simulink subsystem "rss_MotoStallDiaHybr"  (R2023a)
settings: Solver=VariableStepAuto  StartTime=0.0  StopTime=10.0  RelTol=1e-3
undefined symbols (not defined in the file): Cdbl_nElecAgSpdMaxVal, Cdbl_psiPermMagFlxMaxVal, Cdbl_psiPermMagFlxMinVal, ENM_AG_POS_EVAL_MODE, ENM_TYPE_FALT, Gs16_nMotoStallMinRefElecSpd_C, Gu16_ctMotoStallConfCnt_C, Gu16_ctMotoStallRcvyCnt_C, Gu16_psiEstMinPermMagFlx_C
libraries: lib_debounce x1, simulink x1, lib_fault_definiteness x1
settings Model: Creator=xiaoqiang.yuan  LastModifiedBy=xiaoqiang.yuan

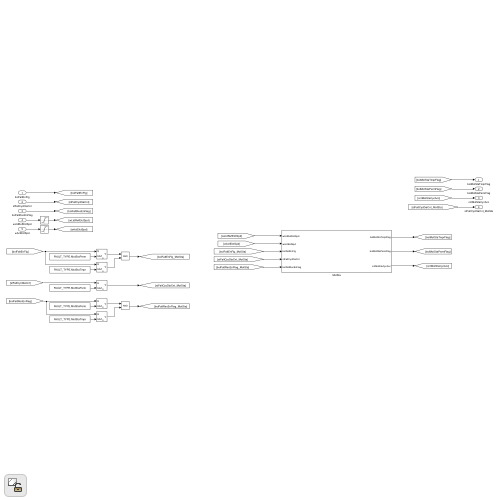
[thumbnail: Simulink's stored preview of the top-level diagram]
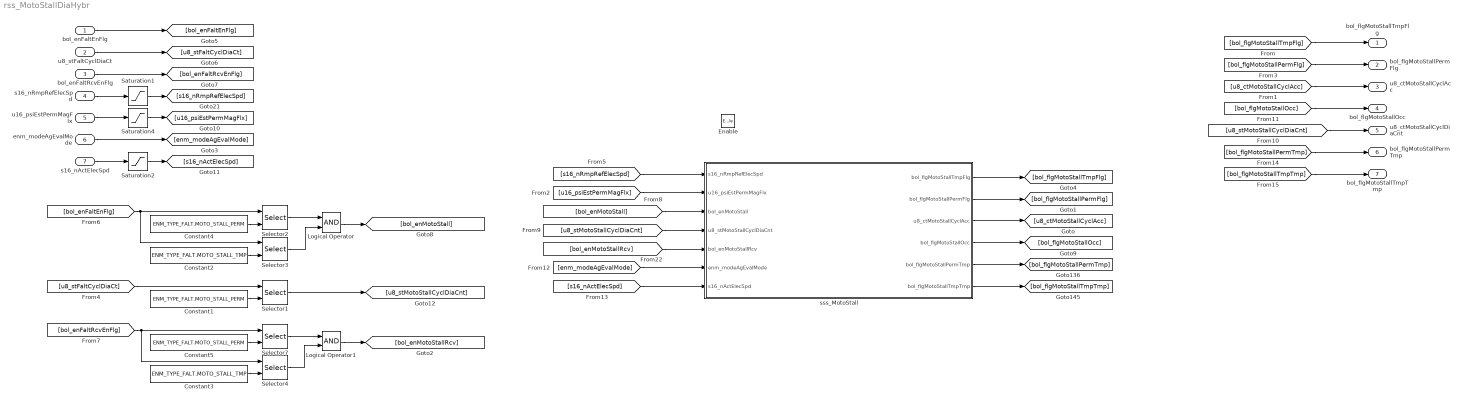
== system rss_MotoStallDiaHybr ==
  bol_enFaltEnFlg : Inport  OutDataTypeStr=boolean
  u8_stFaltCyclDiaCt : Inport  Port=2  OutDataTypeStr=uint8
  bol_enFaltRcvEnFlg : Inport  Port=3  OutDataTypeStr=boolean
  s16_nRmpRefElecSpd : Inport  Port=4  OutDataTypeStr=dt_Standardize_s16p15b0
  u16_psiEstPermMagFlx : Inport  Port=5  OutDataTypeStr=dt_Standardize_u16p15b0
  enm_modeAgEvalMode : Inport  Port=6  OutDataTypeStr=Enum: ENM_AG_POS_EVAL_MODE
  s16_nActElecSpd : Inport  Port=7  OutDataTypeStr=dt_Standardize_s16p15b0
  Enable : EnablePort
  Constant1 : Constant  Value=ENM_TYPE_FALT.MOTO_STALL_PERM
  Constant2 : Constant  Value=ENM_TYPE_FALT.MOTO_STALL_TMP
  Constant3 : Constant  Value=ENM_TYPE_FALT.MOTO_STALL_TMP
  Constant4 : Constant  Value=ENM_TYPE_FALT.MOTO_STALL_PERM
  Constant5 : Constant  Value=ENM_TYPE_FALT.MOTO_STALL_PERM
  Logical Operator : Logic  AllPortsSameDT=off  OutDataTypeStr=boolean
  Logical Operator1 : Logic  AllPortsSameDT=off  OutDataTypeStr=boolean
  Saturation1 : Saturate  UpperLimit=Cdbl_nElecAgSpdMaxVal  LowerLimit=-Cdbl_nElecAgSpdMaxVal
  Saturation2 : Saturate  UpperLimit=Cdbl_nElecAgSpdMaxVal  LowerLimit=-Cdbl_nElecAgSpdMaxVal
  Saturation4 : Saturate  UpperLimit=Cdbl_psiPermMagFlxMaxVal  LowerLimit=Cdbl_psiPermMagFlxMinVal
  Selector{1..4,7} (5 alike) : Selector  IndexMode=Zero-based  InputPortWidth=Cdbl_numFaltDiaNum  IndexOptions=Index vector (port)  Indices=[1 3]  OutputSizes=1
  sss_MotoStall : Subsystem
  bol_flgMotoStallTmpFlg : Outport  OutDataTypeStr=boolean
  bol_flgMotoStallPermFlg : Outport  Port=2  OutDataTypeStr=boolean
  u8_ctMotoStallCyclAcc : Outport  Port=3  OutDataTypeStr=uint8
  bol_flgMotoStallOcc : Outport  Port=4  OutDataTypeStr=boolean
  u8_ctMotoStallCyclDiaCnt : Outport  Port=5  OutDataTypeStr=uint8
  bol_flgMotoStallPermTmp : Outport  Port=6  OutDataTypeStr=boolean
  bol_flgMotoStallTmpTmp : Outport  Port=7  OutDataTypeStr=boolean
  wires:
  [bol_flgMotoStallTmpFlg] -> bol_flgMotoStallTmpFlg/1
  [u8_ctMotoStallCyclAcc] -> u8_ctMotoStallCyclAcc/1
  u8_stFaltCyclDiaCt/1 -> [u8_stFaltCyclDiaCt]
  [bol_enFaltRcvEnFlg] -> Selector7/1, Selector4/1
  s16_nRmpRefElecSpd/1 -> Saturation1/1
  [u8_stMotoStallCyclDiaCnt] -> sss_MotoStall/4(u8_stMotoStallCyclDiaCnt)
  Constant4/1 -> Selector2/2
  Constant5/1 -> Selector7/2
  Selector1/1 -> [u8_stMotoStallCyclDiaCnt]
  sss_MotoStall/1(bol_flgMotoStallTmpFlg) -> [bol_flgMotoStallTmpFlg]
  Constant1/1 -> Selector1/2
  bol_enFaltEnFlg/1 -> [bol_enFaltEnFlg]
  [bol_enMotoStallRcv] -> sss_MotoStall/5(bol_enMotoStallRcv)
  [s16_nRmpRefElecSpd] -> sss_MotoStall/1(s16_nRmpRefElecSpd)
  [bol_enMotoStall] -> sss_MotoStall/3(bol_enMotoStall)
  [bol_enFaltEnFlg] -> Selector2/1, Selector3/1
  [u8_stFaltCyclDiaCt] -> Selector1/1
  bol_enFaltRcvEnFlg/1 -> [bol_enFaltRcvEnFlg]
  [u16_psiEstPermMagFlx] -> sss_MotoStall/2(u16_psiEstPermMagFlx)
  sss_MotoStall/3(u8_ctMotoStallCyclAcc) -> [u8_ctMotoStallCyclAcc]
  sss_MotoStall/2(bol_flgMotoStallPermFlg) -> [bol_flgMotoStallPermFlg]
  [bol_flgMotoStallPermFlg] -> bol_flgMotoStallPermFlg/1
  Constant2/1 -> Selector3/2
  Selector2/1 -> Logical Operator/1
  Selector3/1 -> Logical Operator/2
  Logical Operator/1 -> [bol_enMotoStall]
  Constant3/1 -> Selector4/2
  Selector7/1 -> Logical Operator1/1
  Selector4/1 -> Logical Operator1/2
  Logical Operator1/1 -> [bol_enMotoStallRcv]
  [u8_stMotoStallCyclDiaCnt] -> u8_ctMotoStallCyclDiaCnt/1
  Saturation1/1 -> [s16_nRmpRefElecSpd]
  sss_MotoStall/4(bol_flgMotoStallOcc) -> [bol_flgMotoStallOcc]
  [bol_flgMotoStallOcc] -> bol_flgMotoStallOcc/1
  u16_psiEstPermMagFlx/1 -> Saturation4/1
  Saturation4/1 -> [u16_psiEstPermMagFlx]
  enm_modeAgEvalMode/1 -> [enm_modeAgEvalMode]
  Saturation2/1 -> [s16_nActElecSpd]
  s16_nActElecSpd/1 -> Saturation2/1
  [enm_modeAgEvalMode] -> sss_MotoStall/6(enm_modeAgEvalMode)
  [s16_nActElecSpd] -> sss_MotoStall/7(s16_nActElecSpd)
  [bol_flgMotoStallPermTmp] -> bol_flgMotoStallPermTmp/1
  [bol_flgMotoStallTmpTmp] -> bol_flgMotoStallTmpTmp/1
  sss_MotoStall/5(bol_flgMotoStallPermTmp) -> [bol_flgMotoStallPermTmp]
  sss_MotoStall/6(bol_flgMotoStallTmpTmp) -> [bol_flgMotoStallTmpTmp]

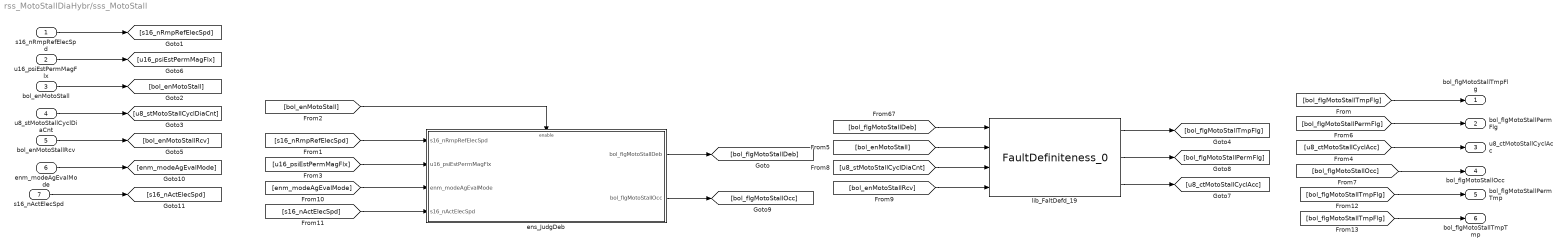
== system rss_MotoStallDiaHybr/sss_MotoStall ==
  s16_nRmpRefElecSpd : Inport
  u16_psiEstPermMagFlx : Inport  Port=2
  bol_enMotoStall : Inport  Port=3
  u8_stMotoStallCyclDiaCnt : Inport  Port=4
  bol_enMotoStallRcv : Inport  Port=5
  enm_modeAgEvalMode : Inport  Port=6
  s16_nActElecSpd : Inport  Port=7
  ens_JudgDeb : Subsystem
  lib_FaltDefd_19 : lib_fault_definiteness/FaultDefiniteness_0  lb_FaltWaitRecvCnt=Gu16_ctMotoStallConfCnt_C
  bol_flgMotoStallTmpFlg : Outport
  bol_flgMotoStallPermFlg : Outport  Port=2
  u8_ctMotoStallCyclAcc : Outport  Port=3
  bol_flgMotoStallOcc : Outport  Port=4
  bol_flgMotoStallPermTmp : Outport  Port=5
  bol_flgMotoStallTmpTmp : Outport  Port=6
  wires:
  [bol_flgMotoStallTmpFlg] -> bol_flgMotoStallTmpTmp/1
  [bol_flgMotoStallTmpFlg] -> bol_flgMotoStallPermTmp/1
  [s16_nActElecSpd] -> ens_JudgDeb/4(s16_nActElecSpd)
  s16_nActElecSpd/1 -> [s16_nActElecSpd]
  [enm_modeAgEvalMode] -> ens_JudgDeb/3(enm_modeAgEvalMode)
  enm_modeAgEvalMode/1 -> [enm_modeAgEvalMode]
  [bol_flgMotoStallOcc] -> bol_flgMotoStallOcc/1
  ens_JudgDeb/2(bol_flgMotoStallOcc) -> [bol_flgMotoStallOcc]
  [u16_psiEstPermMagFlx] -> ens_JudgDeb/2(u16_psiEstPermMagFlx)
  lib_FaltDefd_19/2 -> [bol_flgMotoStallPermFlg]
  [bol_flgMotoStallPermFlg] -> bol_flgMotoStallPermFlg/1
  lib_FaltDefd_19/3 -> [u8_ctMotoStallCyclAcc]
  lib_FaltDefd_19/1 -> [bol_flgMotoStallTmpFlg]
  [u8_ctMotoStallCyclAcc] -> u8_ctMotoStallCyclAcc/1
  u16_psiEstPermMagFlx/1 -> [u16_psiEstPermMagFlx]
  [bol_enMotoStall] -> ens_JudgDeb/Enable
  [s16_nRmpRefElecSpd] -> ens_JudgDeb/1(s16_nRmpRefElecSpd)
  ens_JudgDeb/1(bol_flgMotoStallDeb) -> [bol_flgMotoStallDeb]
  bol_enMotoStallRcv/1 -> [bol_enMotoStallRcv]
  u8_stMotoStallCyclDiaCnt/1 -> [u8_stMotoStallCyclDiaCnt]
  bol_enMotoStall/1 -> [bol_enMotoStall]
  [bol_flgMotoStallTmpFlg] -> bol_flgMotoStallTmpFlg/1
  s16_nRmpRefElecSpd/1 -> [s16_nRmpRefElecSpd]
  [bol_enMotoStallRcv] -> lib_FaltDefd_19/4
  [u8_stMotoStallCyclDiaCnt] -> lib_FaltDefd_19/3
  [bol_enMotoStall] -> lib_FaltDefd_19/2
  [bol_flgMotoStallDeb] -> lib_FaltDefd_19/1

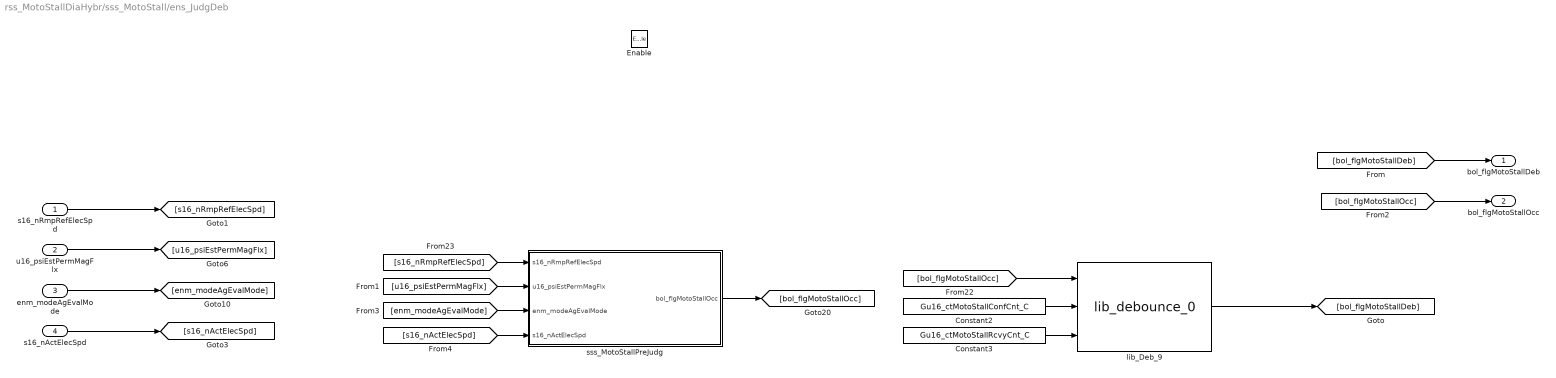
== system rss_MotoStallDiaHybr/sss_MotoStall/ens_JudgDeb ==
  s16_nRmpRefElecSpd : Inport
  u16_psiEstPermMagFlx : Inport  Port=2
  enm_modeAgEvalMode : Inport  Port=3
  s16_nActElecSpd : Inport  Port=4
  Enable : EnablePort
  Constant2 : Constant  Value=Gu16_ctMotoStallConfCnt_C
  Constant3 : Constant  Value=Gu16_ctMotoStallRcvyCnt_C
  lib_Deb_9 : lib_debounce/lib_debounce_0
  sss_MotoStallPreJudg : Subsystem
  bol_flgMotoStallDeb : Outport
  bol_flgMotoStallOcc : Outport  Port=2
  wires:
  [s16_nActElecSpd] -> sss_MotoStallPreJudg/4(s16_nActElecSpd)
  s16_nActElecSpd/1 -> [s16_nActElecSpd]
  [enm_modeAgEvalMode] -> sss_MotoStallPreJudg/3(enm_modeAgEvalMode)
  enm_modeAgEvalMode/1 -> [enm_modeAgEvalMode]
  [bol_flgMotoStallOcc] -> bol_flgMotoStallOcc/1
  [u16_psiEstPermMagFlx] -> sss_MotoStallPreJudg/2(u16_psiEstPermMagFlx)
  u16_psiEstPermMagFlx/1 -> [u16_psiEstPermMagFlx]
  [s16_nRmpRefElecSpd] -> sss_MotoStallPreJudg/1(s16_nRmpRefElecSpd)
  s16_nRmpRefElecSpd/1 -> [s16_nRmpRefElecSpd]
  [bol_flgMotoStallDeb] -> bol_flgMotoStallDeb/1
  sss_MotoStallPreJudg/1(bol_flgMotoStallOcc) -> [bol_flgMotoStallOcc]
  Constant3/1 -> lib_Deb_9/3
  [bol_flgMotoStallOcc] -> lib_Deb_9/1
  lib_Deb_9/1 -> [bol_flgMotoStallDeb]
  Constant2/1 -> lib_Deb_9/2

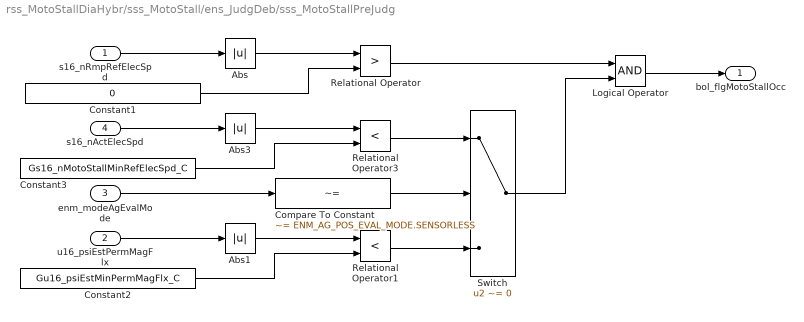
== system rss_MotoStallDiaHybr/sss_MotoStall/ens_JudgDeb/sss_MotoStallPreJudg ==
  s16_nRmpRefElecSpd : Inport
  u16_psiEstPermMagFlx : Inport  Port=2
  enm_modeAgEvalMode : Inport  Port=3
  s16_nActElecSpd : Inport  Port=4
  Abs : Abs  SaturateOnIntegerOverflow=off
  Abs1 : Abs  SaturateOnIntegerOverflow=off
  Abs3 : Abs  SaturateOnIntegerOverflow=off
  Compare To Constant : simulink/Logic and Bit Operations/Compare To Constant  relop=~=  const=ENM_AG_POS_EVAL_MODE.SENSORLESS  OutDataTypeStr=boolean
  Constant1 : Constant  Value=0  OutDataTypeStr=dt_Standardize_s16p15b0
  Constant2 : Constant  Value=Gu16_psiEstMinPermMagFlx_C
  Constant3 : Constant  Value=Gs16_nMotoStallMinRefElecSpd_C
  Logical Operator : Logic  AllPortsSameDT=off  OutDataTypeStr=boolean
  Relational Operator : RelationalOperator  Operator=>  OutDataTypeStr=boolean  RndMeth=Simplest  InputSameDT=off
  Relational Operator1 : RelationalOperator  Operator=<  OutDataTypeStr=boolean  RndMeth=Simplest  InputSameDT=off
  Relational Operator3 : RelationalOperator  Operator=<  OutDataTypeStr=boolean  RndMeth=Simplest  InputSameDT=off
  Switch : Switch  Criteria=u2 ~= 0  SaturateOnIntegerOverflow=off  InputSameDT=off
  bol_flgMotoStallOcc : Outport
  wires:
  Switch/1 -> Logical Operator/2
  Relational Operator1/1 -> Switch/3
  Compare To Constant/1 -> Switch/2
  Relational Operator3/1 -> Switch/1
  enm_modeAgEvalMode/1 -> Compare To Constant/1
  s16_nActElecSpd/1 -> Abs3/1
  Abs3/1 -> Relational Operator3/1
  Constant3/1 -> Relational Operator3/2
  Abs1/1 -> Relational Operator1/1
  Abs/1 -> Relational Operator/1
  Logical Operator/1 -> bol_flgMotoStallOcc/1
  Relational Operator/1 -> Logical Operator/1
  Constant2/1 -> Relational Operator1/2
  u16_psiEstPermMagFlx/1 -> Abs1/1
  Constant1/1 -> Relational Operator/2
  s16_nRmpRefElecSpd/1 -> Abs/1
